simulink model "block_diagram_model"  (R2022a)
settings: Solver=VariableStepAuto  StartTime=0.0  StopTime=10.0  RelTol=1e-3
settings Model: Creator=prafu  LastModifiedBy=prafu

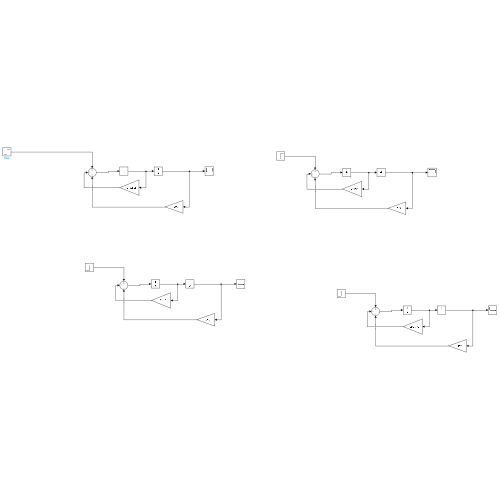
[thumbnail: Simulink's stored preview of the top-level diagram]
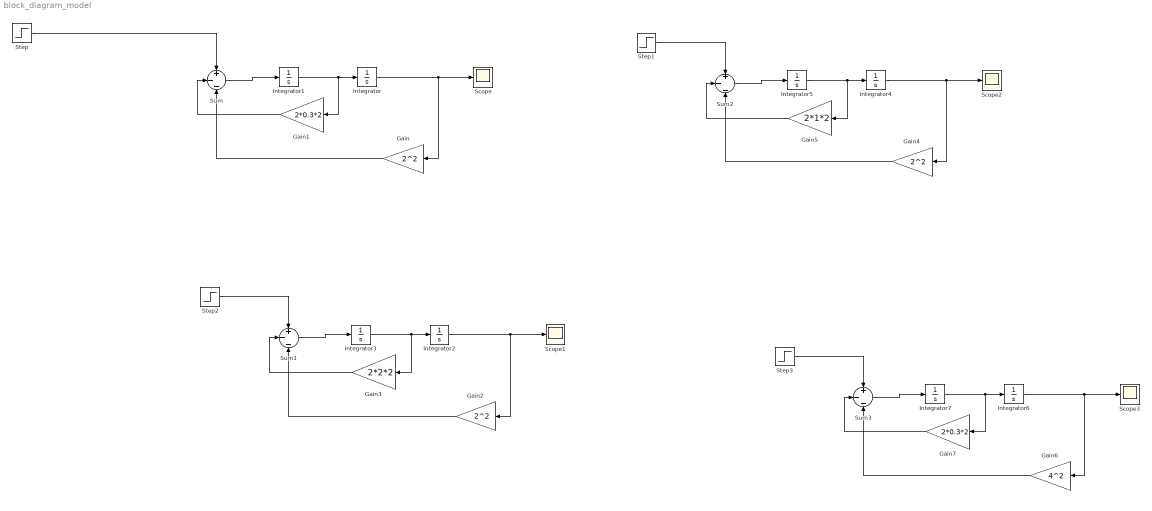
== system block_diagram_model ==
  Gain : Gain  Gain=2^2
  Gain1 : Gain  Gain=2*0.3*2
  Gain2 : Gain  Gain=2^2
  Gain3 : Gain  Gain=2*2*2
  Gain4 : Gain  Gain=2^2
  Gain5 : Gain  Gain=2*1*2
  Gain6 : Gain  Gain=4^2
  Gain7 : Gain  Gain=2*0.3*2
  Integrator{,1..7} (8 alike) : Integrator
  Scope{,1..3} (4 alike) : Scope
  Step{,1..3} (4 alike) : Step  SampleTime=0
  Sum{,1..3} (4 alike) : Sum  Inputs=+|-|-
  wires:
  Sum/1 -> Integrator1/1
  Integrator1/1 -> Gain1/1, Integrator/1
  Integrator/1 -> Scope/1, Gain/1
  Gain/1 -> Sum/3
  Gain1/1 -> Sum/2
  Step1/1 -> Sum2/1
  Sum2/1 -> Integrator5/1
  Integrator5/1 -> Gain5/1, Integrator4/1
  Integrator4/1 -> Scope2/1, Gain4/1
  Gain5/1 -> Sum2/2
  Gain4/1 -> Sum2/3
  Step2/1 -> Sum1/1
  Sum1/1 -> Integrator3/1
  Integrator3/1 -> Gain3/1, Integrator2/1
  Integrator2/1 -> Scope1/1, Gain2/1
  Gain3/1 -> Sum1/2
  Gain2/1 -> Sum1/3
  Step3/1 -> Sum3/1
  Sum3/1 -> Integrator7/1
  Integrator7/1 -> Gain7/1, Integrator6/1
  Integrator6/1 -> Scope3/1, Gain6/1
  Gain7/1 -> Sum3/2
  Gain6/1 -> Sum3/3
  Step/1 -> Sum/1
